simulink model "testharness"  (R2023a)
settings: Solver=ode4  StartTime=0.0  StopTime=30  FixedStep=sim.sample_time_s  RelTol=1e-3
undefined symbols (not defined in the file): rot_K_meas_OB_B_radDs, sfor_meas_B_mDs2, sim
libraries: lib_kinematics x2, simulink x1, matrix_library x1
settings Model: PauseTimes=1  Creator=FC_dev1  LastModifiedBy=FC_dev1

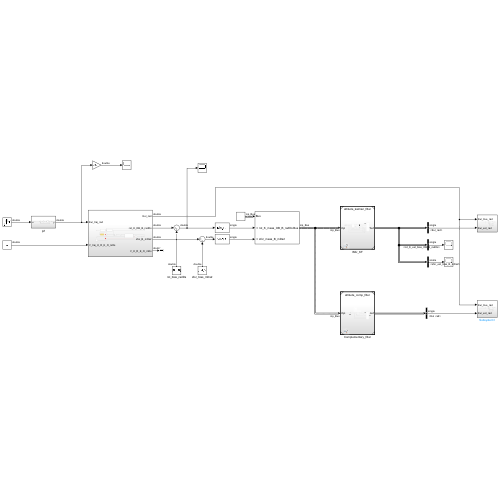
[thumbnail: Simulink's stored preview of the top-level diagram]
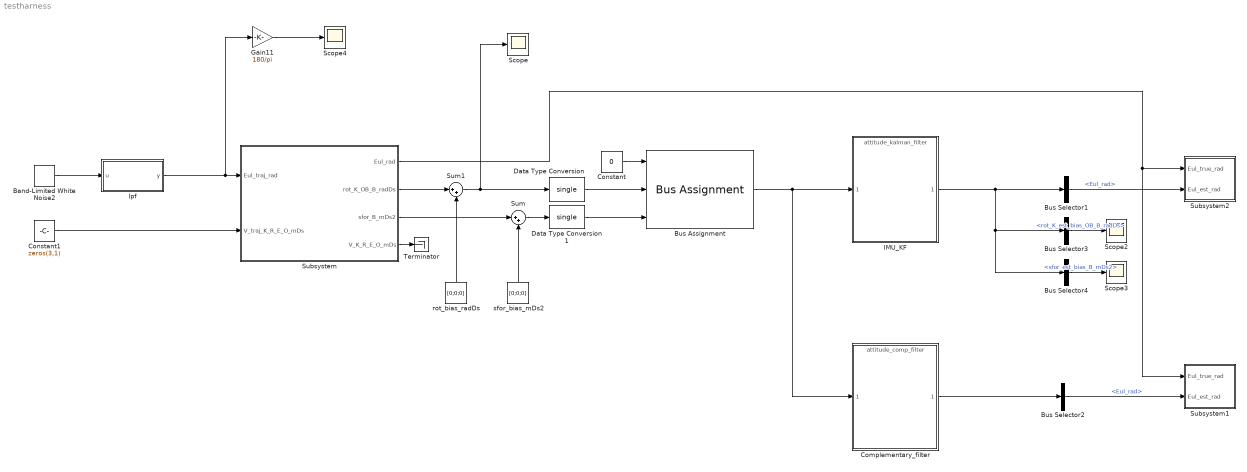
== system testharness ==
  Band-Limited White Noise2 : simulink/Sources/Band-Limited White Noise  Cov=[0.01 0.01 0.01]  Ts=sim.sample_time_s  seed=[23341 23342 23343]
  Bus Assignment : BusAssignment  AssignedSignals=rot_K_meas_OB_B_radDs,sfor_meas_B_mDs2
  Bus Selector1 : BusSelector  OutputSignals=Eul_rad
  Bus Selector2 : BusSelector  OutputSignals=Eul_rad
  Bus Selector3 : BusSelector  OutputSignals=rot_K_est_bias_OB_B_radDs
  Bus Selector4 : BusSelector  OutputSignals=sfor_est_bias_B_mDs2
  Complementary_filter : ModelReference  ModelNameDialog=attitude_comp_filter.slx  SimulationMode=Normal  ModelReferenceVersion=1.195
  Constant : Constant  Value=0  OutDataTypeStr=Bus: inp_Bus
  Constant1 : Constant  Value=zeros(3,1)  VectorParams1D=off
  Data Type Conversion : DataTypeConversion  OutDataTypeStr=single  SaturateOnIntegerOverflow=off  RndMeth=Floor
  Data Type Conversion1 : DataTypeConversion  OutDataTypeStr=single  SaturateOnIntegerOverflow=off  RndMeth=Floor
  Gain11 : Gain  Gain=180/pi
  IMU_KF : ModelReference  ModelNameDialog=attitude_kalman_filter.slx  SimulationMode=Normal  ModelReferenceVersion=1.202
  Scope{,2..4} (4 alike) : Scope
  Subsystem : Subsystem
  Subsystem1 : Subsystem
  Subsystem2 : Subsystem
  Sum : Sum  Inputs=|++
  Sum1 : Sum  Inputs=|++
  Terminator : Terminator
  lpf : Subsystem
  rot_bias_radDs : Constant  Value=[0;0;0]  VectorParams1D=off
  sfor_bias_mDs2 : Constant  Value=[0;0;0]  VectorParams1D=off
  wires:
  Constant/1 -> Bus Assignment/1
  Bus Assignment/1 -> Complementary_filter/1, IMU_KF/1
  Data Type Conversion/1 -> Bus Assignment/2
  Data Type Conversion1/1 -> Bus Assignment/3
  Subsystem/1(Eul_rad) -> Subsystem1/1(Eul_true_rad), Subsystem2/1(Eul_true_rad)
  Subsystem/2(rot_K_OB_B_radDs) -> Sum1/1
  Subsystem/3(sfor_B_mDs2) -> Sum/1
  IMU_KF/1 -> Bus Selector3/1, Bus Selector4/1, Bus Selector1/1
  Bus Selector1/1 -> Subsystem2/2(Eul_est_rad)  "<Eul_rad>"
  Bus Selector3/1 -> Scope2/1  "<rot_K_est_bias_OB_B_radDs>"
  Bus Selector4/1 -> Scope3/1  "<sfor_est_bias_B_mDs2>"
  Band-Limited White Noise2/1 -> lpf/1(u)
  Gain11/1 -> Scope4/1
  Constant1/1 -> Subsystem/2(V_traj_K_R_E_O_mDs)
  Subsystem/4(V_K_R_E_O_mDs) -> Terminator/1
  Sum/1 -> Data Type Conversion1/1
  Sum1/1 -> Data Type Conversion/1, Scope/1
  rot_bias_radDs/1 -> Sum1/2
  sfor_bias_mDs2/1 -> Sum/2
  lpf/1(y) -> Gain11/1, Subsystem/1(Eul_traj_rad)
  Complementary_filter/1 -> Bus Selector2/1
  Bus Selector2/1 -> Subsystem1/2(Eul_est_rad)  "<Eul_rad>"

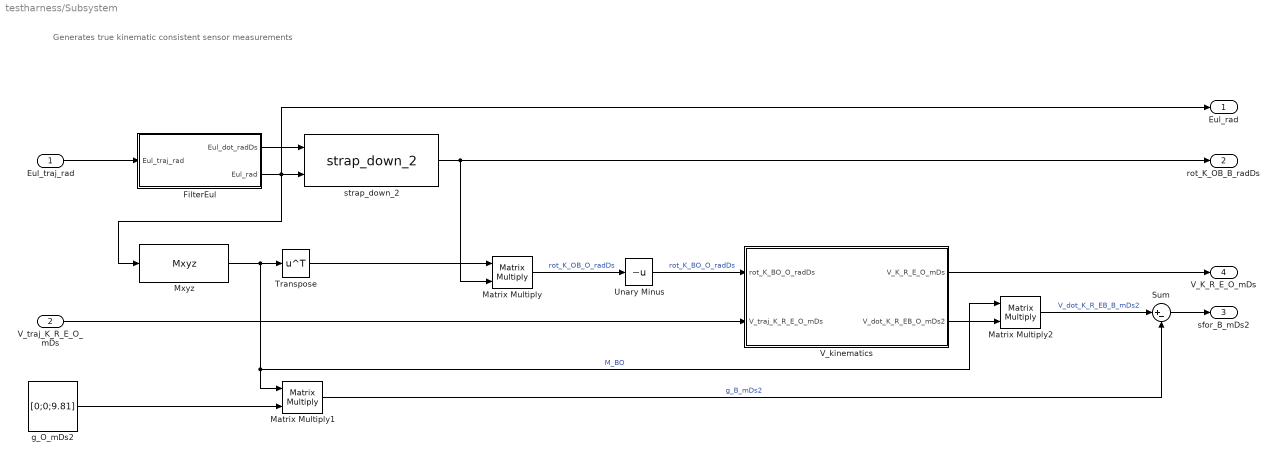
== system testharness/Subsystem ==
  note: Generates true kinematic consistent sensor measurements
  Eul_traj_rad : Inport
  V_traj_K_R_E_O_mDs : Inport  Port=2
  FilterEul : Subsystem
  Matrix Multiply : Product  Multiplication=Matrix(*)
  Matrix Multiply1 : Product  Multiplication=Matrix(*)
  Matrix Multiply2 : Product  Multiplication=Matrix(*)
  Mxyz : lib_kinematics/Mxyz  SystemSampleTime=-1  VariantActivationTime=update diagram  Latency=0  AutoFrameSizeCalculation=off
  Sum : Sum  Inputs=|+-
  Transpose : Math  Operator=transpose
  Unary Minus : UnaryMinus
  V_kinematics : Subsystem
  g_O_mDs2 : Constant  Value=[0;0;9.81]  VectorParams1D=off
  strap_down_2 : lib_kinematics/strap_down_2  SystemSampleTime=-1  VariantActivationTime=update diagram  Latency=0  AutoFrameSizeCalculation=off
  Eul_rad : Outport
  rot_K_OB_B_radDs : Outport  Port=2
  sfor_B_mDs2 : Outport  Port=3
  V_K_R_E_O_mDs : Outport  Port=4
  wires:
  Eul_traj_rad/1 -> FilterEul/1(Eul_traj_rad)
  V_traj_K_R_E_O_mDs/1 -> V_kinematics/2(V_traj_K_R_E_O_mDs)
  FilterEul/1(Eul_dot_radDs) -> strap_down_2/1
  FilterEul/2(Eul_rad) -> Mxyz/1, Eul_rad/1, strap_down_2/2
  Mxyz/1 -> Matrix Multiply2/1, Matrix Multiply1/1, Transpose/1  "M_BO"
  Transpose/1 -> Matrix Multiply/1
  strap_down_2/1 -> rot_K_OB_B_radDs/1, Matrix Multiply/2
  Matrix Multiply/1 -> Unary Minus/1  "rot_K_OB_O_radDs"
  Unary Minus/1 -> V_kinematics/1(rot_K_BO_O_radDs)  "rot_K_BO_O_radDs"
  g_O_mDs2/1 -> Matrix Multiply1/2
  Matrix Multiply1/1 -> Sum/2  "g_B_mDs2"
  Sum/1 -> sfor_B_mDs2/1
  V_kinematics/2(V_dot_K_R_EB_O_mDs2) -> Matrix Multiply2/2
  Matrix Multiply2/1 -> Sum/1  "V_dot_K_R_EB_B_mDs2"
  V_kinematics/1(V_K_R_E_O_mDs) -> V_K_R_E_O_mDs/1

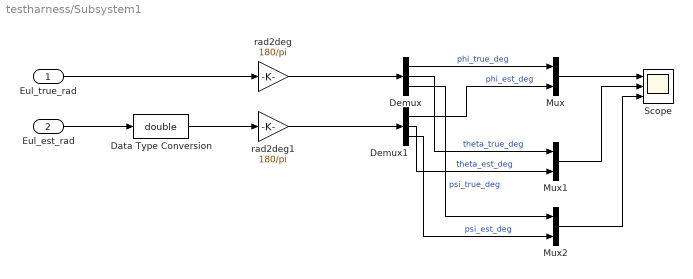
== system testharness/Subsystem1 ==
  Eul_true_rad : Inport
  Eul_est_rad : Inport  Port=2
  Data Type Conversion : DataTypeConversion  OutDataTypeStr=double  SaturateOnIntegerOverflow=off  RndMeth=Floor
  Demux : Demux  Outputs=3
  Demux1 : Demux  Outputs=3
  Mux : Mux  Inputs=2
  Mux1 : Mux  Inputs=2
  Mux2 : Mux  Inputs=2
  Scope : Scope  NumInputPorts=3
  rad2deg : Gain  Gain=180/pi  OutDataTypeStr=Inherit: Same as input
  rad2deg1 : Gain  Gain=180/pi  OutDataTypeStr=Inherit: Same as input
  wires:
  Eul_est_rad/1 -> Data Type Conversion/1
  Eul_true_rad/1 -> rad2deg/1
  rad2deg/1 -> Demux/1
  rad2deg1/1 -> Demux1/1
  Demux/1 -> Mux/1  "phi_true_deg"
  Demux1/1 -> Mux/2  "phi_est_deg"
  Demux/2 -> Mux1/1  "theta_true_deg"
  Demux1/2 -> Mux1/2  "theta_est_deg"
  Demux/3 -> Mux2/1  "psi_true_deg"
  Demux1/3 -> Mux2/2  "psi_est_deg"
  Mux/1 -> Scope/1
  Mux1/1 -> Scope/2
  Mux2/1 -> Scope/3
  Data Type Conversion/1 -> rad2deg1/1

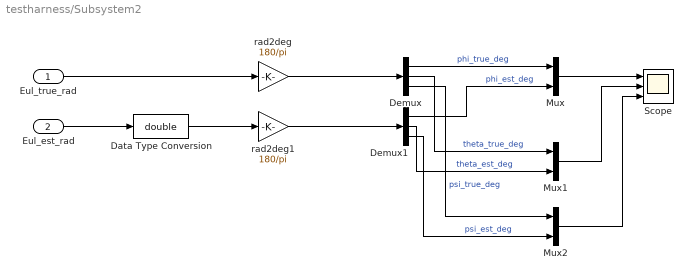
== system testharness/Subsystem2 ==
  Eul_true_rad : Inport
  Eul_est_rad : Inport  Port=2
  Data Type Conversion : DataTypeConversion  OutDataTypeStr=double  SaturateOnIntegerOverflow=off  RndMeth=Floor
  Demux : Demux  Outputs=3
  Demux1 : Demux  Outputs=3
  Mux : Mux  Inputs=2
  Mux1 : Mux  Inputs=2
  Mux2 : Mux  Inputs=2
  Scope : Scope  NumInputPorts=3
  rad2deg : Gain  Gain=180/pi  OutDataTypeStr=Inherit: Same as input
  rad2deg1 : Gain  Gain=180/pi  OutDataTypeStr=Inherit: Same as input
  wires:
  Data Type Conversion/1 -> rad2deg1/1
  Mux2/1 -> Scope/3
  Mux1/1 -> Scope/2
  Mux/1 -> Scope/1
  Demux1/3 -> Mux2/2  "psi_est_deg"
  Demux/3 -> Mux2/1  "psi_true_deg"
  Demux1/2 -> Mux1/2  "theta_est_deg"
  Demux/2 -> Mux1/1  "theta_true_deg"
  Demux1/1 -> Mux/2  "phi_est_deg"
  Demux/1 -> Mux/1  "phi_true_deg"
  rad2deg1/1 -> Demux1/1
  rad2deg/1 -> Demux/1
  Eul_true_rad/1 -> rad2deg/1
  Eul_est_rad/1 -> Data Type Conversion/1

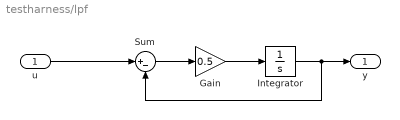
== system testharness/lpf ==
  u : Inport
  Gain : Gain  Gain=0.5
  Integrator : Integrator
  Sum : Sum  Inputs=|+-
  y : Outport
  wires:
  u/1 -> Sum/1
  Sum/1 -> Gain/1
  Gain/1 -> Integrator/1
  Integrator/1 -> Sum/2, y/1

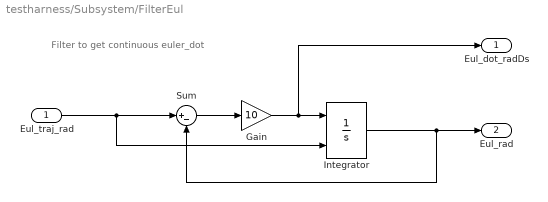
== system testharness/Subsystem/FilterEul ==
  note: Filter to get continuous euler_dot
  Eul_traj_rad : Inport
  Gain : Gain  Gain=10
  Integrator : Integrator  InitialConditionSource=external
  Sum : Sum  Inputs=|+-
  Eul_dot_radDs : Outport
  Eul_rad : Outport  Port=2
  wires:
  Eul_traj_rad/1 -> Integrator/2, Sum/1
  Sum/1 -> Gain/1
  Gain/1 -> Eul_dot_radDs/1, Integrator/1
  Integrator/1 -> Sum/2, Eul_rad/1

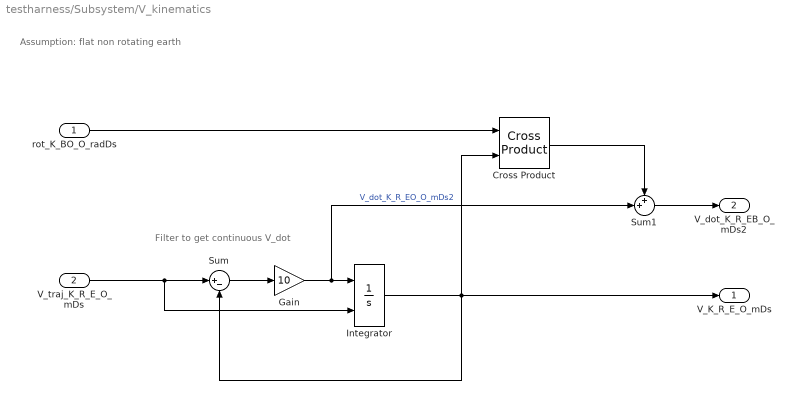
== system testharness/Subsystem/V_kinematics ==
  note: Assumption: flat non rotating earth
  note: Filter to get continuous V_dot
  rot_K_BO_O_radDs : Inport
  V_traj_K_R_E_O_mDs : Inport  Port=2
  Cross Product : matrix_library/Cross Product
  Gain : Gain  Gain=10
  Integrator : Integrator  InitialConditionSource=external
  Sum : Sum  Inputs=|+-
  Sum1 : Sum  Inputs=++|
  V_K_R_E_O_mDs : Outport
  V_dot_K_R_EB_O_mDs2 : Outport  Port=2
  wires:
  V_traj_K_R_E_O_mDs/1 -> Sum/1, Integrator/2
  Sum/1 -> Gain/1
  Gain/1 -> Sum1/2, Integrator/1  "V_dot_K_R_EO_O_mDs2"
  Integrator/1 -> Cross Product/2, Sum/2, V_K_R_E_O_mDs/1
  rot_K_BO_O_radDs/1 -> Cross Product/1
  Sum1/1 -> V_dot_K_R_EB_O_mDs2/1
  Cross Product/1 -> Sum1/1
